simulink model "untitled"  (R2019b)
settings: Solver=VariableStepAuto  StartTime=0.0  StopTime=0.5  RelTol=1e-3
libraries: dsparch4 x1
settings Model: Creator=Dell  LastModifiedBy=Dell

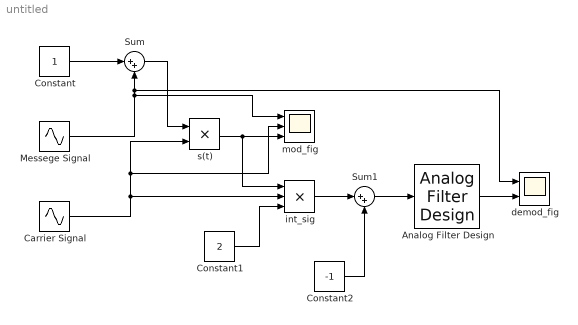
== system untitled ==
  Analog Filter Design : dsparch4/Analog Filter Design  method=Butterworth  filttype=Lowpass  N=8  Wlo=2*pi*13  Whi=80  Rp=2  Rs=40
  Carrier Signal : Sin  Frequency=2*pi*200  Phase=pi/2  SampleTime=1/10000
  Constant : Constant
  Constant1 : Constant  Value=2
  Constant2 : Constant  Value=-1
  "Messege Signal " : Sin  Amplitude=2  Frequency=2*pi*10  SampleTime=1/10000
  Sum : Sum  Inputs=|++
  Sum1 : Sum  Inputs=|++
  "demod_fig " : Scope  NumInputPorts=2
  "int_sig " : Product  Inputs=3
  "mod_fig " : Scope  NumInputPorts=3
  s(t) : Product
  wires:
  "Messege Signal "/1 -> "demod_fig "/1, Sum/2, "mod_fig "/1
  Sum/1 -> s(t)/1
  Constant/1 -> Sum/1
  s(t)/1 -> "int_sig "/1, "mod_fig "/3
  Carrier Signal/1 -> "mod_fig "/2, s(t)/2, "int_sig "/2
  Constant1/1 -> "int_sig "/3
  "int_sig "/1 -> Sum1/1
  Constant2/1 -> Sum1/2
  Sum1/1 -> Analog Filter Design/1
  Analog Filter Design/1 -> "demod_fig "/2
